simulink model "param_ident_online"  (R2025b)
settings: Solver=VariableStepAuto  StartTime=0.0  StopTime=40  RelTol=1e-3
InitFcn:
  | rng('shuffle')
  | Cl_delta_low = 0.5;
  | Cl_delta_high = 2.5;
  | C0_mean = 0.1;
  | C0_bound = 0;
  | C0_low = C0_mean - C0_bound;
  | C0_high = C0_mean + C0_bound;
  | Cl_delta_delay = 0.6;
  | C0_delay = 0.3;
libraries: simulink x4
settings Model: Creator=finnb  LastModifiedBy=trist

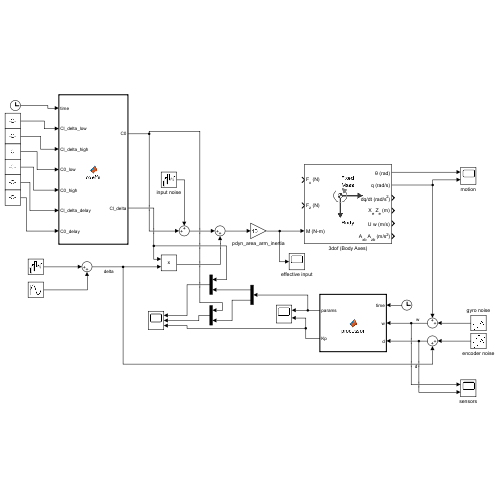
[thumbnail: Simulink's stored preview of the top-level diagram]
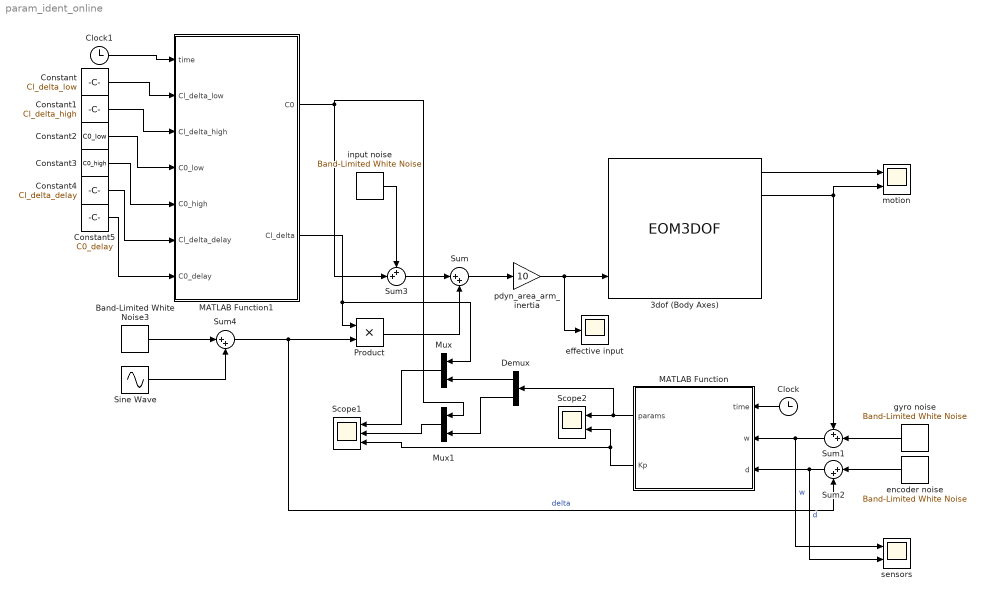
== system param_ident_online ==
  3dof (Body Axes) : EOM3DOF
  Band-Limited White Noise3 : simulink/Sources/Band-Limited White Noise  Cov=[1e-2]  Ts=0.03  seed=[23341]
  Clock : Clock
  Clock1 : Clock
  Constant : Constant  Value=Cl_delta_low
  Constant1 : Constant  Value=Cl_delta_high
  Constant2 : Constant  Value=C0_low
  Constant3 : Constant  Value=C0_high
  Constant4 : Constant  Value=Cl_delta_delay
  Constant5 : Constant  Value=C0_delay
  Demux : Demux  Outputs=2
  MATLAB Function : MATLAB Function  TreatAsAtomicUnit=on
  MATLAB Function1 : MATLAB Function  TreatAsAtomicUnit=on  SystemSampleTime=0.01
  Mux : Mux  Inputs=2
  Mux1 : Mux  Inputs=2
  Product : Product
  Scope1 : Scope  NumInputPorts=3
      settings: ActiveDisplayYMinimum=0.0078190731743709163  ActiveDisplayYMaximum=2.9496487877000455  DataLoggingVariableName=ScopeData4
  Scope2 : Scope  NumInputPorts=2
      settings: ActiveDisplayYMinimum=-1  ActiveDisplayYMaximum=1  DataLoggingVariableName=ScopeData2
  Sine Wave : Sin  Frequency=10  Phase=pi/2  SampleTime=0
  Sum : Sum  Inputs=|++
  Sum1 : Sum  Inputs=++|
  Sum2 : Sum  Inputs=|++
  Sum3 : Sum  Inputs=++|
  Sum4 : Sum  Inputs=|++
  effective input : Scope
      settings: ActiveDisplayYMinimum=-109.33479965380702  ActiveDisplayYMaximum=113.50306593607439
  encoder noise : simulink/Sources/Band-Limited White Noise  Cov=[1e-6]  Ts=0.01  seed=[23341]
  gyro noise : simulink/Sources/Band-Limited White Noise  Cov=[1e-7]  Ts=0.01  seed=[23341]
  input noise : simulink/Sources/Band-Limited White Noise  Cov=[1e-6]  Ts=0.2  seed=[23341]
  motion : Scope  NumInputPorts=2
      settings: ActiveDisplayYMinimum=-3.9240694878775417  ActiveDisplayYMaximum=3.9237328145742758
  pdyn_area_arm_inertia : Gain  Gain=10
  sensors : Scope  NumInputPorts=2
      settings: ActiveDisplayYMinimum=-0.021581740856872682  ActiveDisplayYMaximum=0.046913425503183052  DataLoggingVariableName=ScopeData3
  wires:
  Sum4/1 -> Product/2, Sum2/2  "delta"
  3dof (Body Axes)/2 -> Sum1/1, motion/2
  Clock/1 -> MATLAB Function/1(time)
  MATLAB Function/1(params) -> Demux/1, Scope2/1
  Sum1/1 -> sensors/1, MATLAB Function/2(w)  "w"
  gyro noise/1 -> Sum1/2
  Sum2/1 -> sensors/2, MATLAB Function/3(d)  "d"
  encoder noise/1 -> Sum2/1
  input noise/1 -> Sum3/1
  pdyn_area_arm_inertia/1 -> effective input/1, 3dof (Body Axes)/3
  Band-Limited White Noise3/1 -> Sum4/1
  Sine Wave/1 -> Sum4/2
  3dof (Body Axes)/1 -> motion/1
  MATLAB Function/2(Kp) -> Scope2/2, Scope1/3
  Sum/1 -> pdyn_area_arm_inertia/1
  Sum3/1 -> Sum/1
  Product/1 -> Sum/2
  MATLAB Function1/2(Cl_delta) -> Product/1, Mux/1
  MATLAB Function1/1(C0) -> Mux1/1, Sum3/2
  Clock1/1 -> MATLAB Function1/1(time)
  Demux/1 -> Mux/2
  Mux/1 -> Scope1/1
  Demux/2 -> Mux1/2
  Mux1/1 -> Scope1/2
  Constant/1 -> MATLAB Function1/2(Cl_delta_low)
  Constant1/1 -> MATLAB Function1/3(Cl_delta_high)
  Constant2/1 -> MATLAB Function1/4(C0_low)
  Constant3/1 -> MATLAB Function1/5(C0_high)
  Constant4/1 -> MATLAB Function1/6(Cl_delta_delay)
  Constant5/1 -> MATLAB Function1/7(C0_delay)

== matlab function param_ident_online/MATLAB Function1 ==
  data: C0 output; time input; Cl_delta output; Cl_delta_low input; Cl_delta_high input; C0_low input; C0_high input; Cl_delta_delay input; C0_delay input
function [C0, Cl_delta] = coeffs(time, Cl_delta_low, Cl_delta_high, C0_low, C0_high, Cl_delta_delay, C0_delay)
    t = time/40.0;
    Cl_delta = Cl_delta_low + (Cl_delta_high - Cl_delta_low) / (1 + exp(-10*(t - Cl_delta_delay)));
    C0 = C0_low + (C0_high - C0_low) / (1 + exp(-10*(t - C0_delay)));
end

== matlab function param_ident_online/MATLAB Function ==
  settings: updateMethod=DISCRETE  sampleTime=0.005
  data: time input; w input; params output; d input; Kp output
function [params, Kp] = processor(time, w, d)
    % p : parameters
    % r : regressors
    % w : angular rate measurement
    % d : canard angle measurement / command

    pdyn_area_arm_inertia = 10; % everything in L except coefficients. match with gain in sim
    if abs(d) < 0.01
        d = 0;
    end

    [params, Kp] = param_estimator_kf(time, w, d, pdyn_area_arm_inertia);

end
